simulink model "egr560_tracking_sim"  (R2025b)
settings: Solver=FixedStepDiscrete  StartTime=0.0  StopTime=Tsim  FixedStep=Ts  RelTol=1e-3
values from neighbouring files (symbols this model uses):
  Ad = sysd.A    [main_baseline.m]
  Bd = sysd.B(:,1)    [main_baseline.m]
  Bplant = [Bd Ed]    [main_baseline.m]
  delta_max = 0.5    [main_baseline.m]
  delta_rate_max = 0.5    [main_baseline.m]
  Dplant = zeros(4,2)    [main_baseline.m]
  Ed = sysd.B(:,2)    [main_baseline.m]
  M_wmax = 50    [main_baseline.m]
  sigma_meas = 5e-5    (= 5e-05)    [main_baseline.m]
  Ts = 0.02    [main_baseline.m]
  wheelbase = lf + lr    (= 2.6)    [main_baseline.m]
undefined symbols (not defined in the file or in its folder): K
settings Model: Creator=prajj  LastModifiedBy=prajj
settings DataIOCC: ReturnWorkspaceOutputs=off

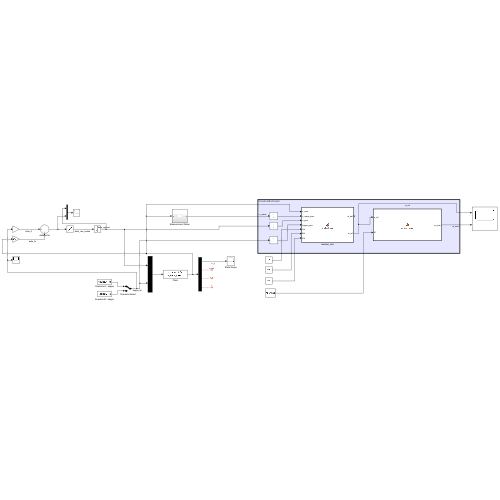
[thumbnail: Simulink's stored preview of the top-level diagram]
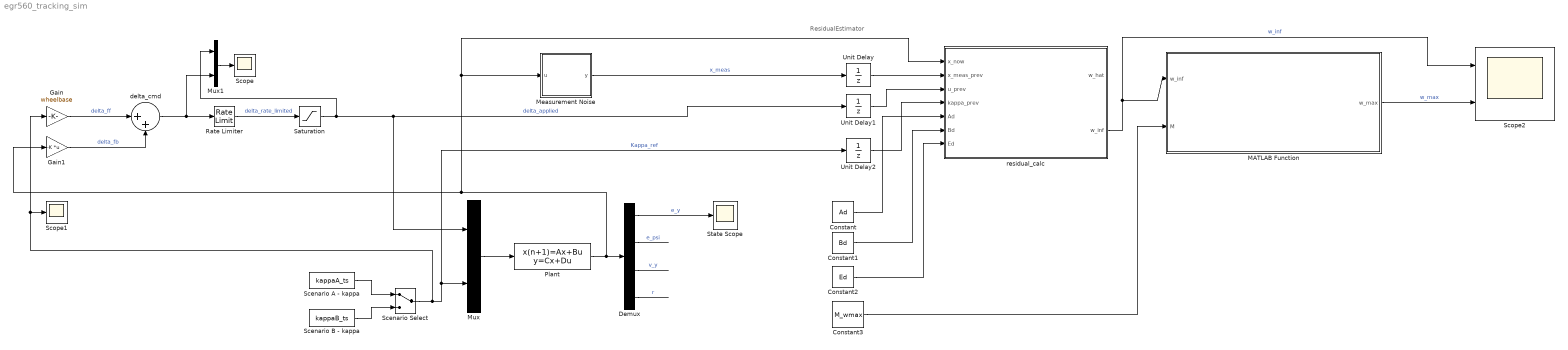
== system egr560_tracking_sim ==
  note: ResidualEstimator
  Constant : Constant  Value=Ad
  Constant1 : Constant  Value=Bd
  Constant2 : Constant  Value=Ed
  Constant3 : Constant  Value=M_wmax
  Demux : Demux
  Gain : Gain  Gain=wheelbase
  Gain1 : Gain  Gain=-K  Multiplication=Matrix(K*u)
  MATLAB Function : MATLAB Function  TreatAsAtomicUnit=on
  Measurement Noise : Subsystem
  Mux : Mux  Inputs=2
  Mux1 : Mux  Inputs=2
  Plant : DiscreteStateSpace  A=Ad  B=Bplant  C=eye(4)  D=Dplant  InitialCondition=[0;0;0;0]  SampleTime=Ts
  Rate Limiter : RateLimiter  RisingSlewLimit=delta_rate_max  FallingSlewLimit=-delta_rate_max  SampleTimeMode=inherited
  Saturation : Saturate  UpperLimit=delta_max  LowerLimit=-delta_max
  Scenario A - kappa : FromWorkspace  VariableName=kappaA_ts
  Scenario B - kappa : FromWorkspace  VariableName=kappaB_ts
  Scenario Select : ManualSwitch
  Scope : Scope
      settings: ActiveDisplayYMinimum=-1  ActiveDisplayYMaximum=1  DataLoggingVariableName=ScopeData2
  Scope1 : Scope
      settings: ActiveDisplayYMinimum=-1  ActiveDisplayYMaximum=1
  Scope2 : Scope  NumInputPorts=2
      settings: ActiveDisplayYMinimum=-2.6707711315674575E-5  ActiveDisplayYMaximum=0.00024036940184107123  DataLoggingVariableName=ScopeData3
  State Scope : Scope
      settings: ActiveDisplayYMinimum=-0.0043967747622156812  ActiveDisplayYMaximum=0.000489753109930898
  Unit Delay : UnitDelay  InitialCondition=[0;0;0;0]  SampleTime=Ts  HasFrameUpgradeWarning=on
  Unit Delay1 : UnitDelay  SampleTime=Ts  HasFrameUpgradeWarning=on
  Unit Delay2 : UnitDelay  SampleTime=Ts  HasFrameUpgradeWarning=on
  delta_cmd : Sum  Inputs=|++
  residual_calc : MATLAB Function  TreatAsAtomicUnit=on
  wires:
  Scenario A - kappa/1 -> Scenario Select/1
  Scenario B - kappa/1 -> Scenario Select/2
  Scenario Select/1 -> Unit Delay2/1, Mux/2, Gain/1, Scope1/1  "Kappa_ref"
  Mux/1 -> Plant/1
  Plant/1 -> residual_calc/1(x_now), Measurement Noise/1(u), Gain1/1, Demux/1
  Demux/1 -> State Scope/1  "e_y"
  Demux/2 -> ?  "e_psi"
  Demux/3 -> ?  "v_y"
  Demux/4 -> ?  "r"
  Gain/1 -> delta_cmd/1  "delta_ff"
  Gain1/1 -> delta_cmd/2  "delta_fb"
  delta_cmd/1 -> Mux1/2, Rate Limiter/1
  Mux1/1 -> Scope/1
  Rate Limiter/1 -> Saturation/1  "delta_rate_limited"
  Saturation/1 -> Unit Delay1/1, Mux/1, Mux1/1  "delta_applied"
  Measurement Noise/1(y) -> Unit Delay/1  "x_meas"
  Unit Delay2/1 -> residual_calc/4(kappa_prev)
  Unit Delay1/1 -> residual_calc/3(u_prev)
  Unit Delay/1 -> residual_calc/2(x_meas_prev)
  Constant/1 -> residual_calc/5(Ad)
  Constant1/1 -> residual_calc/6(Bd)
  Constant2/1 -> residual_calc/7(Ed)
  Constant3/1 -> MATLAB Function/2(M)
  residual_calc/2(w_inf) -> Scope2/1, MATLAB Function/1(w_inf)  "w_inf"
  MATLAB Function/1(w_max) -> Scope2/2  "w_max"

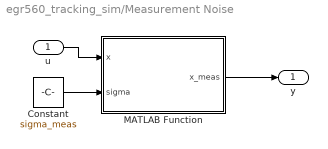
== system egr560_tracking_sim/Measurement Noise ==
  u : Inport
  Constant : Constant  Value=sigma_meas
  MATLAB Function : MATLAB Function  TreatAsAtomicUnit=on
  y : Outport
  wires:
  u/1 -> MATLAB Function/1(x)
  MATLAB Function/1(x_meas) -> y/1
  Constant/1 -> MATLAB Function/2(sigma)

== matlab function egr560_tracking_sim/residual_calc ==
  data: x_now input; w_hat output; x_meas_prev input; u_prev input; kappa_prev input; Ad input; Bd input; Ed input; w_inf output
function [w_hat, w_inf] = residual_calc(x_now, x_meas_prev, u_prev, kappa_prev, Ad, Bd, Ed)
x_pred = Ad*x_meas_prev + Bd*u_prev + Ed*kappa_prev;
w_hat = x_now - x_pred;
w_inf = max(abs(w_hat));

== matlab function egr560_tracking_sim/Measurement Noise/MATLAB Function ==
  data: x input; x_meas output; sigma input
function x_meas = add_noise(x, sigma)
x_meas = x + sigma*randn(4,1);

== matlab function egr560_tracking_sim/MATLAB Function ==
  data: w_inf input; w_max output; M input
function w_max = rolling_max(w_inf, M)
persistent buf idx filled

if isempty(buf)
    buf = zeros(1,M);
    idx = 1;
    filled = 0;
end

buf(idx) = w_inf;
idx = idx + 1;
if idx > M
    idx = 1;
end

if filled < M
    filled = filled + 1;
end

w_max = max(buf(1:filled));
